simulink model "Exercise1"  (Simulink 7.2)
settings: Solver=ode45  StartTime=0.0  StopTime=10.0  RelTol=1e-3
undefined symbols (not defined in the file): b, k, m
settings Model: Creator=Inderjot  LastModifiedBy=Inderjot

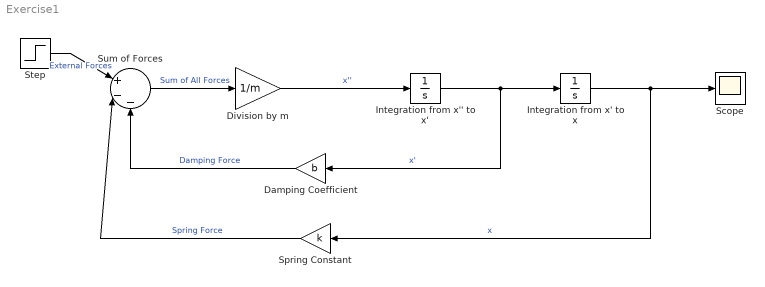
== system Exercise1 ==
  Damping Coefficient : Gain  Orientation=left  Gain=b  ParameterDataType=sfix(16)  ParameterScaling=2^0  OutDataType=sfix(16)  OutScaling=2^0
  Division by m : Gain  Gain=1/m  ParameterDataType=sfix(16)  ParameterScaling=2^0  OutDataType=sfix(16)  OutScaling=2^0
  Integration from x' to x : Integrator
  Integration from x'' to x' : Integrator
  Scope : Scope
  Spring Constant : Gain  Orientation=left  Gain=k  ParameterDataType=sfix(16)  ParameterScaling=2^0  OutDataType=sfix(16)  OutScaling=2^0
  Step : Step  Time=0  After=4  SampleTime=0
  Sum of Forces : Sum  Inputs=|+--  OutDataType=sfix(16)  OutScaling=2^0
  wires:
  Integration from x'' to x'/1 -> Integration from x' to x/1, Damping Coefficient/1  "x'"
  Division by m/1 -> Integration from x'' to x'/1  "x''"
  Integration from x' to x/1 -> Spring Constant/1, Scope/1  "x"
  Damping Coefficient/1 -> Sum of Forces/3  "Damping Force"
  Spring Constant/1 -> Sum of Forces/2  "Spring Force"
  Step/1 -> Sum of Forces/1  "External Forces"
  Sum of Forces/1 -> Division by m/1  "Sum of All Forces"
